simulink model "BLDC_Hysteresis_Speed_Current_Loop"  (R2022b)
settings: Solver=FixedStepDiscrete  StartTime=0.0  StopTime=2  FixedStep=1e-5  RelTol=1e-3
libraries: spsPermanentMagnetSynchronousMachineLib x1, spsDCVoltageSourceLib x1, slpidlib x1, spsTwoLevelConverterLib x1, spspowerguiLib x1
settings Model: Creator=31904  LastModifiedBy=31904

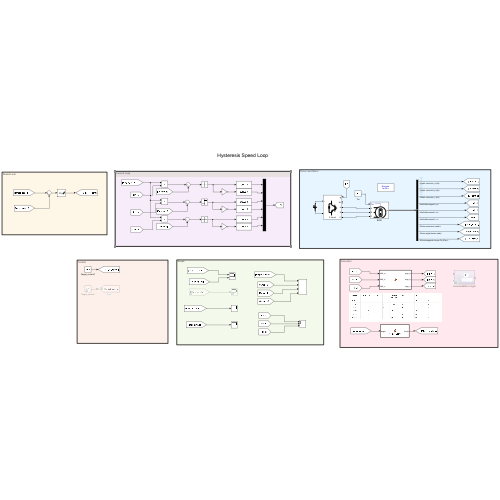
[thumbnail: Simulink's stored preview of the top-level diagram]
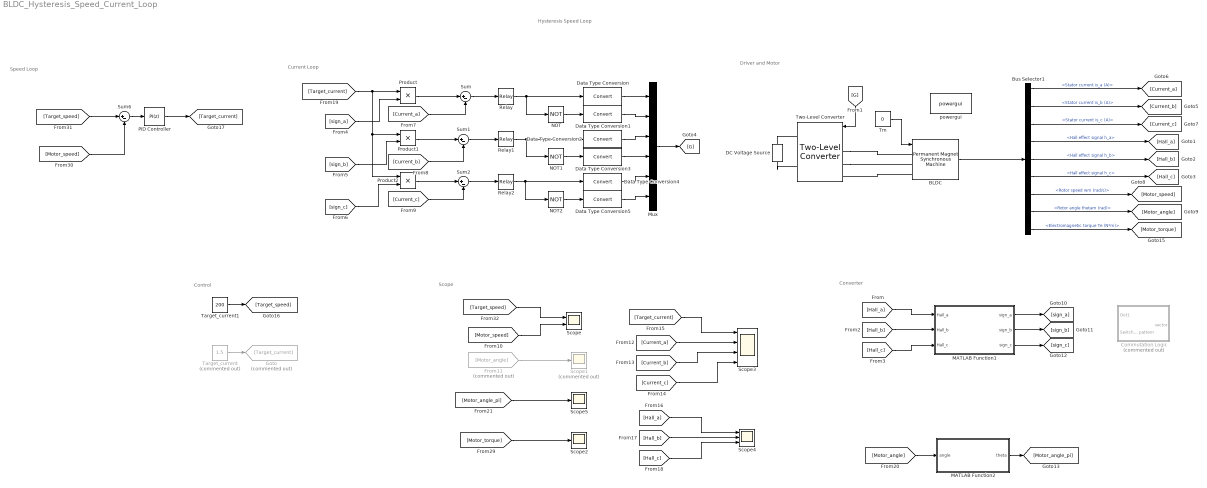
== system BLDC_Hysteresis_Speed_Current_Loop ==
  note: Converter
  note: Speed Loop
  note: Current Loop
  note: Control
  note: Scope
  note: Hysteresis Speed Loop
  note: Driver and Motor
  BLDC : spsPermanentMagnetSynchronousMachineLib/Permanent Magnet Synchronous Machine  NbPhases=3  FluxDistribution=Trapezoidal  RotorType=Round  MechanicalLoad=Torque Tm  PresetModel=No  ShowDetailedParameters=on  MeasurementBus=off  Resistance=0.0485  Inductance=8.5e-3  dqInductances=[8.5e-3,8.5e-3]  La=0.000395  MachineConstant=Flux linkage established by magnets (V.s)  Flux=0.1194  VoltageCst=50.0142  TorqueCst=0.4776  Flat=120  Mechanical=[0.0027 0.0004924 2 0]  PolePairs=4  InitialConditions=[0,0, 0,0]  InitialConditions5ph=[0 0 0 0 0 0]  RefAngle=Aligned with phase A axis (original Park)  IterativeDiscreteModel=Trapezoidal non iterative  TsBlock=-1  TsPowergui=0
  Bus Selector1 : BusSelector  OutputSignals=Stator current is_a (A),Stator current is_b (A),Stator current is_c (A),Hall effect signal h_a,Hall effect signal h_b,Hall effect signal h_c,Rotor speed wm (rad/s),Rotor angle thetam (rad),Electromagnetic torque Te (N*m)
  Commutation Logic : Subsystem  Commented=on
  DC Voltage Source : spsDCVoltageSourceLib/DC Voltage Source  Amplitude=60  Measurements=None
  Data Type Conversion{,1..5} (6 alike) : DataTypeConversion  SaturateOnIntegerOverflow=off  RndMeth=Floor
  From11 : From  Commented=on  GotoTag=Motor_angle
  Goto : Goto  Commented=on  GotoTag=Target_current
  MATLAB Function1 : MATLAB Function  TreatAsAtomicUnit=on
  MATLAB Function2 : MATLAB Function  TreatAsAtomicUnit=on
  Mux : Mux  Inputs=6
  NOT : Logic  Operator=NOT  IconShape=distinctive  AllPortsSameDT=off  OutDataTypeStr=boolean
  NOT1 : Logic  Operator=NOT  IconShape=distinctive  AllPortsSameDT=off  OutDataTypeStr=boolean
  NOT2 : Logic  Operator=NOT  IconShape=distinctive  AllPortsSameDT=off  OutDataTypeStr=boolean
  PID Controller : slpidlib/PID Controller  Controller=PI  Form=Parallel  TimeDomain=Discrete-time  UseExternalTs=off  SampleTime=-1  IntegratorMethod=Forward Euler  FilterMethod=Forward Euler  ControllerParametersSource=internal  P=1  I=1.1  UseKiTs=off  D=0  N=100  UseFilter=on  TunerSelectOption=Transfer Function Based (PID Tuner App)  InitialConditionSource=internal  InitialConditionForIntegrator=0  InitialConditionForFilter=0  DifferentiatorICPrevScaledInput=0  ExternalReset=none  TrackingMode=off  Kt=1  LimitOutput=on  SatLimitsSource=internal  UpperSaturationLimit=20  LowerSaturationLimit=0  LinearizeAsGain=on  AntiWindupMode=none  Kb=1  LimitIntegrator=off  UpperIntegratorSaturationLimit=inf  LowerIntegratorSaturationLimit=-inf  POutMin=[]  POutMax=[]  IOutMin=[]  IOutMax=[]  DOutMin=[]  DOutMax=[]  NOutMin=[]  NOutMax=[]  SumOutMin=[]  SumOutMax=[]  SaturationOutMin=[]  SaturationOutMax=[]  PParamMin=[]  PParamMax=[]  IParamMin=[]  IParamMax=[]  DParamMin=[]  DParamMax=[]  NParamMin=[]  NParamMax=[]  KbParamMin=[]  KbParamMax=[]  KtParamMin=[]  KtParamMax=[]  KbOutMin=[]  KbOutMax=[]  KtOutMin=[]  KtOutMax=[]  IntegratorOutMin=[]  IntegratorOutMax=[]  FilterOutMin=[]  FilterOutMax=[]  SumI1OutMin=[]  SumI1OutMax=[]  SumI2OutMin=[]  SumI2OutMax=[]  SumI3OutMin=[]  SumI3OutMax=[]  SumI4OutMin=[]  SumI4OutMax=[]  SumDOutMin=[]  SumDOutMax=[]  DifferentiatorOutMin=[]  DifferentiatorOutMax=[]  FilterDiffOutCoefMin=[]  FilterDiffOutCoefMax=[]  ReciprocalOutMin=[]  ReciprocalOutMax=[]  SumDenOutMin=[]  SumDenOutMax=[]  SumNumOutMin=[]  SumNumOutMax=[]  DivideOutMin=[]  DivideOutMax=[]  UdiffTsProdOutMin=[]  UdiffTsProdOutMax=[]  NTsProdOutMin=[]  NTsProdOutMax=[]  UintegralTsProdOutMin=[]  UintegralTsProdOutMax=[]  UngainTsProdOutMin=[]  UngainTsProdOutMax=[]  ClampingZeroOutDataTypeStr=Inherit: Inherit via back propagation  ClampingZeroOutMin=[]  ClampingZeroOutMax=[]  FilterDenConstantOutDataTypeStr=Inherit: Inherit via back propagation  FilterDenConstantOutMin=[]  FilterDenConstantOutMax=[]  PCopyOutDataTypeStr=Inherit: Inherit via back propagation  PCopyOutMin=[]  PCopyOutMax=[]  NCopyOutDataTypeStr=Inherit: Inherit via back propagation  NCopyOutMin=[]  NCopyOutMax=[]  IntegratorContinuousStateAttributes=''  IntegratorStateMustResolveToSignalObject=off  IntegratorRTWStateStorageClass=Auto  FilterContinuousStateAttributes=''  FilterStateMustResolveToSignalObject=off  FilterRTWStateStorageClass=Auto  ParallelPVariant=InternalParameters  IdealPVariant=Disabled  IVariant=InternalParameters  DVariant=Disabled  IntegratorVariant=Discrete  SatVariant=Enabled  AWVariant=Passthrough  PCopyVariant=Disabled  TRVariant=Disabled  FdbkBlocksVariant=Forward  IdealPFdbkVariant=Disabled  SatFdbkVariant=Disabled  DerivativeFilterVariant=Disabled  NVariant=Disabled  NCopyVariant=Disabled_SignalSpec  FilterICVariant=Disabled  IntegratorICVariant=InternalICs  ExternalResetVariant=Disabled  TRSumVariant=Passthrough  SumFdbkVariant=Disabled  SumVariant=Sum_PI  TsampFilterVariant=InternalTs  TsampNgainVariant=Passthrough  TsampIntegralVariant=Passthrough  ExternalSaturationOutDataTypeStr=Inherit: Same as second input
  Product : Product
  Product1 : Product
  Product2 : Product
  Relay : Relay  OnSwitchValue=0.1  OffSwitchValue=-0.1
  Relay1 : Relay  OnSwitchValue=0.1  OffSwitchValue=-0.1
  Relay2 : Relay  OnSwitchValue=0.1  OffSwitchValue=-0.1
  Scope : Scope  NumInputPorts=2
  Scope1 : Scope  Commented=on
  Scope2 : Scope
  Scope3 : Scope  NumInputPorts=4
  Scope4 : Scope  NumInputPorts=3
  Scope5 : Scope
  Sum{,1..2,6} (4 alike) : Sum  Inputs=|+-
  Target_current : Constant  Commented=on  Value=1.5
  Target_current1 : Constant  Value=200
  Tm : Constant  Value=0
  Two-Level Converter : spsTwoLevelConverterLib/Two-Level Converter  ModelType=Switching devices  Ron=1e-3  Rs=1e6  Cs=inf  Vforward=[0,0]  Ron_Diode=1e-3  Rs_Diode=1e6  Cs_Diode=inf  Vf_Diode=1e-3  Rs_CurrentSource=inf  Ron_ACsource=1e-3
  powergui : spspowerguiLib/powergui  Priority=1  SimulationMode=Discrete  SampleTime=0.00001  frequency=60  Iterations=50  frequencyindice=0  Pbase=100e6  ErrMax=1e-4  UnitsV=kV  UnitsW=MW  buscounter=0  FunctionMessages=off  echomessages=off  EnableUseOfTLC=off  CurrentSourceSwitches=off  DisableSnubberDevices=off  DisableRonSwitches=off  DisableVfSwitches=off  DisplayEquations=off  AutomaticDiscreteSolvers=off  SolverType=Tustin/Backward Euler (TBE)  Interpol=off  ExternalGateDelay=off  methode=off  Ts=100  x0status=blocks  SPID=on  SwTol=0  HookPort=off  NonlinearTolerance=1e-4  nMaxIteration=100  ContinueOnMaxIteration=off  RestoreLinks=warning  ResistiveCurrentMeasurement=off  Frange=[0:2:500]  Ylog=off  Xlog=on  ShowGrid=off  save=off  variable=ZData  structure=0  ZoomFFT=off  StartTime=0.0  cycles=1  DisplayStyle=1  fundamental=60  FreqAxis=off  MaxFrequency=1000  frequencyindicesteady=1  RmsSteady=1  display=off
  wires:
  Tm/1 -> BLDC/1
  [G] -> Two-Level Converter/1
  Bus Selector1/3 -> [Current_c]  "<Stator current is_c (A)>"
  Bus Selector1/8 -> [Motor_angle]  "<Rotor angle thetam (rad)>"
  Bus Selector1/1 -> [Current_a]  "<Stator current is_a (A)>"
  Bus Selector1/6 -> [Hall_c]  "<Hall effect signal h_c>"
  Bus Selector1/4 -> [Hall_a]  "<Hall effect signal h_a>"
  Bus Selector1/2 -> [Current_b]  "<Stator current is_b (A)>"
  Bus Selector1/7 -> [Motor_speed]  "<Rotor speed wm (rad/s)>"
  Bus Selector1/5 -> [Hall_b]  "<Hall effect signal h_b>"
  BLDC/1 -> Bus Selector1/1
  [Hall_a] -> MATLAB Function1/1(Hall_a)
  [Hall_b] -> MATLAB Function1/2(Hall_b)
  [Hall_c] -> MATLAB Function1/3(Hall_c)
  MATLAB Function1/1(sign_a) -> [sign_a]
  MATLAB Function1/2(sign_b) -> [sign_b]
  MATLAB Function1/3(sign_c) -> [sign_c]
  [Target_current] -> Product2/1, Product1/1, Product/1
  [sign_a] -> Product/2
  [sign_b] -> Product1/2
  [sign_c] -> Product2/2
  Product/1 -> Sum/1
  Product1/1 -> Sum1/1
  Product2/1 -> Sum2/1
  [Current_a] -> Sum/2
  [Current_b] -> Sum1/2
  [Current_c] -> Sum2/2
  Sum/1 -> Relay/1
  Sum1/1 -> Relay1/1
  Sum2/1 -> Relay2/1
  Relay/1 -> Data Type Conversion/1, NOT/1
  NOT/1 -> Data Type Conversion1/1
  NOT1/1 -> Data Type Conversion3/1
  Relay1/1 -> NOT1/1, Data Type Conversion2/1
  NOT2/1 -> Data Type Conversion5/1
  Relay2/1 -> NOT2/1, Data Type Conversion4/1
  Data Type Conversion/1 -> Mux/1
  Data Type Conversion1/1 -> Mux/2
  Data Type Conversion2/1 -> Mux/3
  Data Type Conversion3/1 -> Mux/4
  Data Type Conversion4/1 -> Mux/5
  Data Type Conversion5/1 -> Mux/6
  Mux/1 -> [G]
  [Motor_speed] -> Scope/2
  [Current_a] -> Scope3/2
  [Current_b] -> Scope3/3
  [Current_c] -> Scope3/4
  Target_current/1 -> Goto/1
  [Target_current] -> Scope3/1
  [Hall_a] -> Scope4/1
  [Hall_b] -> Scope4/2
  [Hall_c] -> Scope4/3
  From11/1 -> Scope1/1
  [Motor_angle] -> MATLAB Function2/1(angle)
  [Motor_angle_pi] -> Scope5/1
  MATLAB Function2/1(theta) -> [Motor_angle_pi]
  Bus Selector1/9 -> [Motor_torque]  "<Electromagnetic torque Te (N*m)>"
  [Motor_torque] -> Scope2/1
  [Motor_speed] -> Sum6/2
  Target_current1/1 -> [Target_speed]
  [Target_speed] -> Sum6/1
  Sum6/1 -> PID Controller/1
  PID Controller/1 -> [Target_current]
  [Target_speed] -> Scope/1
  connections:
  Two-Level Converter/LConn2 -- BLDC/LConn2
  BLDC/LConn3 -- Two-Level Converter/LConn3
  Two-Level Converter/LConn1 -- BLDC/LConn1
  DC Voltage Source/LConn1 -- Two-Level Converter/RConn2
  DC Voltage Source/RConn1 -- Two-Level Converter/RConn1

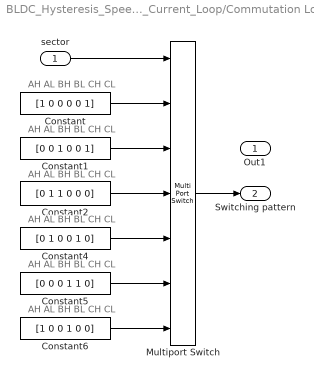
== system BLDC_Hysteresis_Speed_Current_Loop/Commutation Logic ==
  note: AH AL BH BL CH CL
  note: AH AL BH BL CH CL
  note: AH AL BH BL CH CL
  note: AH AL BH BL CH CL
  note: AH AL BH BL CH CL
  note: AH AL BH BL CH CL
  sector : Inport
  Constant : Constant  Value=[1 0 0 0 0 1]
  Constant1 : Constant  Value=[0 0 1 0 0 1]
  Constant2 : Constant  Value=[0 1 1 0 0 0]
  Constant4 : Constant  Value=[0 1 0 0 1 0]
  Constant5 : Constant  Value=[0 0 0 1 1 0]
  Constant6 : Constant  Value=[1 0 0 1 0 0]
  Multiport Switch : MultiPortSwitch  Inputs=6  SaturateOnIntegerOverflow=off  InputSameDT=off
  Out1 : Outport
  "  Switching pattern" : Outport  Port=2  VectorParamsAs1DForOutWhenUnconnected=off
  wires:
  Constant4/1 -> Multiport Switch/5
  Constant5/1 -> Multiport Switch/6
  Constant6/1 -> Multiport Switch/7
  sector/1 -> Multiport Switch/1
  Constant2/1 -> Multiport Switch/4
  Multiport Switch/1 -> "  Switching pattern"/1
  Constant1/1 -> Multiport Switch/3
  Constant/1 -> Multiport Switch/2

== matlab function BLDC_Hysteresis_Speed_Current_Loop/MATLAB Function2 ==
  data: angle input; theta output
function theta = Angle_Conv(angle)

n=mod(angle,pi);

theta = n;

== matlab function BLDC_Hysteresis_Speed_Current_Loop/MATLAB Function1 ==
  data: Hall_a input; sign_a output; Hall_b input; Hall_c input; sign_b output; sign_c output
function [sign_a,sign_b,sign_c] = fcn(Hall_a, Hall_b, Hall_c)

if Hall_a==1&&Hall_b==0&&Hall_c==1

sign_a=1;
sign_b=0;
sign_c=-1;

elseif Hall_a==1&&Hall_b==0&&Hall_c==0

sign_a=0;
sign_b=1;
sign_c=-1;


elseif Hall_a==1&&Hall_b==1&&Hall_c==0

sign_a=-1;
sign_b=1;
sign_c=0;


elseif Hall_a==0&&Hall_b==1&&Hall_c==0

sign_a=-1;
sign_b=0;
sign_c=1;


elseif Hall_a==0&&Hall_b==1&&Hall_c==1

sign_a=0;
sign_b=-1;
sign_c=1;

else

sign_a=1;
sign_b=-1;
sign_c=0;


end
